simulink model "voltage_isochronous_droop_01"  (R2020b)
settings: Solver=VariableStepAuto  StartTime=0.0  StopTime=5  RelTol=1e-3
undefined symbols (not defined in the file): DiscIntNeverNeededParam, droop1, droop2
libraries: fl_lib x14, nesl_utility x9, simulink x1
settings Model: Creator=gdudgeon  LastModifiedBy=gdudgeon

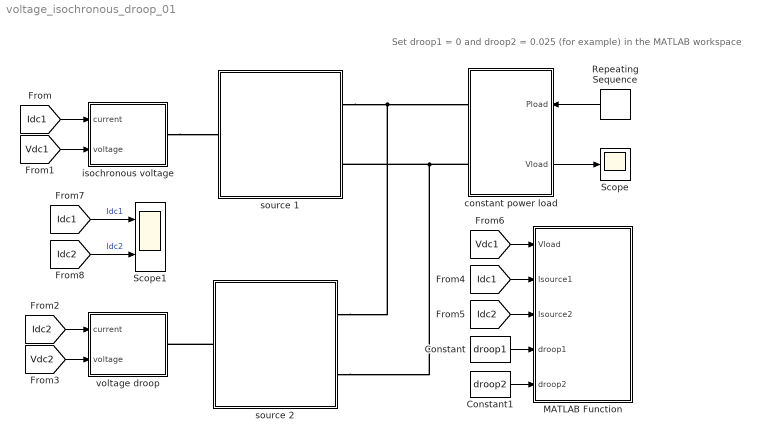
== system voltage_isochronous_droop_01 ==
  note: Set droop1 = 0 and droop2 = 0.025 (for example) in the MATLAB workspace
  Constant : Constant  Value=droop1
  Constant1 : Constant  Value=droop2
  MATLAB Function : MATLAB Function  TreatAsAtomicUnit=on  SystemSampleTime=Tanim  mask(Machine Rotor Animation){Tanim=0.01}
      mask prompts: Tanim "Animation Rate [s]"
      mask help: This block animates permanent magnet inside a stator. The "thetaRotor" input is the angle of the rotor. The "phase" parameter must be defined in the workspace and selects the energized coil in the stator.
  Repeating Sequence : simulink/Sources/Repeating Sequence  rep_seq_t=[0 10 20]  rep_seq_y=[1 1 1]
  Scope : Scope
  Scope1 : Scope  NumInputPorts=2
  constant power load : Subsystem
      settings: PortSchema="{\"entries\":[{\"content\":{\"sides\":[{\"content\":{\"connectorIds\":[\"LConn1\",\"LConn2\"]},\"type\":\"ConnectorPlacement.EquallySpacedRectSide\",\"uuid\":\"ede3b789-4807-48db-8c98-272deebb1f90\"},{\"content\":{\"connectorIds\":[\"In1\",\"Out1\"],\"side\":\"RIGHT\"},\"type\":\"ConnectorPlacement.EquallySpacedRectSide\",\"uuid\":\"cedec5e8-adcb-43e2-ab37-681d5d79ce2a\"},{\"content\":{\"connectorIds\":[],\"side\":\"TOP\"},\"type\":\"ConnectorPlacement.EquallySpacedRectSide\",\"uuid\":\"08b52c53-b13a-4cd2-b8db-308d9ebd4277\"},{\"content\":{\"connectorIds\":[],\"side\":\"HIDDEN\"},\"type\":\"ConnectorPlacement.EquallySpacedRectSide\",\"uuid\":\"3f956204-c540-4879-b053-0f78777aeccb\"}]},\"type\":\"ConnectorPlacement.EquallySpacedConnector\",\"uuid\":\"42303a72-b7ff-4a69-b636-ebca1dcca68c\"}],\"packageUris\":[\"http://schema.mathworks.com/mf0/Connector/R2020b\"],\"version\":\"1.0\"}"
  isochronous voltage : Subsystem  mask{droop=droop1}
  source 1 : Subsystem
  "source 2 " : Subsystem
  voltage droop : Subsystem  mask{droop=droop2}
  wires:
  constant power load/1(Vload) -> Scope/1
  Repeating Sequence/1 -> constant power load/1(Pload)
  Constant/1 -> MATLAB Function/4(droop1)
  Constant1/1 -> MATLAB Function/5(droop2)
  [Idc1] -> isochronous voltage/1(current)
  [Vdc1] -> isochronous voltage/2(voltage)
  [Vdc2] -> voltage droop/2(voltage)
  [Idc2] -> voltage droop/1(current)
  [Idc1] -> MATLAB Function/2(Isource1)
  [Idc2] -> MATLAB Function/3(Isource2)
  [Vdc1] -> MATLAB Function/1(Vload)
  [Idc1] -> Scope1/1  "Idc1"
  [Idc2] -> Scope1/2  "Idc2"
  connections:
  constant power load/LConn2 -- "source 2 "/RConn2 -- source 1/RConn2
  "source 2 "/LConn1 -- voltage droop/RConn1
  source 1/RConn1 -- "source 2 "/RConn1 -- constant power load/LConn1
  isochronous voltage/RConn1 -- source 1/LConn1

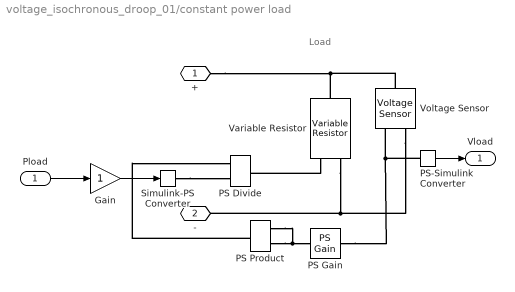
== system voltage_isochronous_droop_01/constant power load ==
  note: Load
  Pload : Inport
  Gain : Gain
  PS Divide : fl_lib/Physical Signals/Functions/PS Divide
      settings: SourceProductBaseCode=SS
  PS Gain : fl_lib/Physical Signals/Functions/PS Gain  gain=-1
  PS Product : fl_lib/Physical Signals/Functions/PS Product
  PS-Simulink Converter : nesl_utility/PS-Simulink Converter  PhysicalDomain=network_engine_domain  SubClassName=ps_output  LeftPortType=input  RightPortType=output  PseudoPeriodic=off  Frequencies=[]  Unit=inherit  AffineConversion=off
  Simulink-PS Converter : nesl_utility/Simulink-PS Converter  PhysicalDomain=network_engine_domain  SubClassName=ps_input  LeftPortType=input  RightPortType=output  PseudoPeriodic=off  Frequencies=[]  NoiseDistribution=none  NoiseParameters=[]  Unit=W  AffineConversion=off  FilteringAndDerivatives=provide  SimscapeFilterOrder=1  InputFilterTimeConstant=0.001  UdotUserProvided=0
  Variable Resistor : fl_lib/Electrical/Electrical Elements/Variable Resistor  Rmin=1 Ohm  i_specify=off  i_priority=None  i=0 A  i_nominal_specify=off  i_nominal_unit=A  i_nominal_value=1  v_specify=off  v_priority=None  v=0 V  v_nominal_specify=off  v_nominal_unit=V  v_nominal_value=1
  Voltage Sensor : fl_lib/Electrical/Electrical Sensors/Voltage Sensor
  + : PMIOPort  Side=Left
  - : PMIOPort  Port=2  Side=Left
  Vload : Outport
  wires:
  PS-Simulink Converter/1 -> Vload/1
  Pload/1 -> Gain/1
  Gain/1 -> Simulink-PS Converter/1
  connections:
  PS-Simulink Converter/LConn1 -- PS Gain/LConn1 -- Voltage Sensor/RConn1
  Variable Resistor/LConn1 -- PS Divide/RConn1
  Voltage Sensor/RConn2 -- -/RConn1 -- Variable Resistor/LConn2
  Voltage Sensor/LConn1 -- +/RConn1 -- Variable Resistor/RConn1
  Simulink-PS Converter/RConn1 -- PS Divide/LConn2
  PS Product/LConn1 -- PS Product/LConn2 -- PS Gain/RConn1
  PS Product/RConn1 -- PS Divide/LConn1

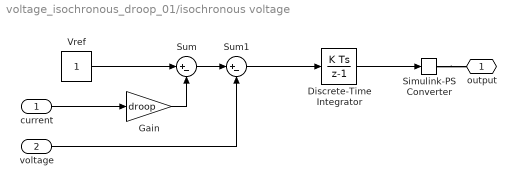
== system voltage_isochronous_droop_01/isochronous voltage ==
  current : Inport
  voltage : Inport  Port=2
  Discrete-Time Integrator : DiscreteIntegrator  gainval=100  InitialCondition=0.5  SampleTime=-1  ICPrevOutput=DiscIntNeverNeededParam  ICPrevScaledInput=DiscIntNeverNeededParam
  Gain : Gain  Gain=droop
  Simulink-PS Converter : nesl_utility/Simulink-PS Converter  PhysicalDomain=network_engine_domain  SubClassName=ps_input  LeftPortType=input  RightPortType=output  PseudoPeriodic=off  Frequencies=[]  NoiseDistribution=none  NoiseParameters=[]  Unit=1  AffineConversion=off  FilteringAndDerivatives=provide  SimscapeFilterOrder=1  InputFilterTimeConstant=0.001  UdotUserProvided=0
  Sum : Sum  Inputs=|+-
  Sum1 : Sum  Inputs=|+-
  Vref : Constant
  output : PMIOPort  Side=Right
  wires:
  voltage/1 -> Sum1/2
  Vref/1 -> Sum/1
  Gain/1 -> Sum/2
  Sum/1 -> Sum1/1
  current/1 -> Gain/1
  Discrete-Time Integrator/1 -> Simulink-PS Converter/1
  Sum1/1 -> Discrete-Time Integrator/1
  connections:
  Simulink-PS Converter/RConn1 -- output/RConn1

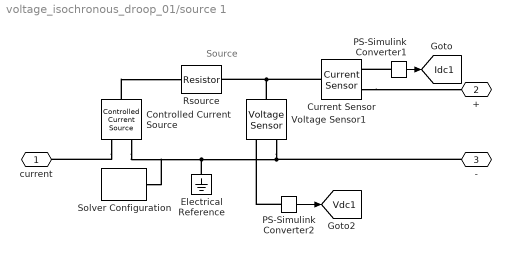
== system voltage_isochronous_droop_01/source 1 ==
  note: Source
  Controlled Current Source : fl_lib/Electrical/Electrical Sources/Controlled Current Source
  Current Sensor : fl_lib/Electrical/Electrical Sensors/Current Sensor
  Electrical Reference : fl_lib/Electrical/Electrical Elements/Electrical Reference
  PS-Simulink Converter1 : nesl_utility/PS-Simulink Converter  PhysicalDomain=network_engine_domain  SubClassName=ps_output  LeftPortType=input  RightPortType=output  PseudoPeriodic=off  Frequencies=[]  Unit=inherit  AffineConversion=off
  PS-Simulink Converter2 : nesl_utility/PS-Simulink Converter  PhysicalDomain=network_engine_domain  SubClassName=ps_output  LeftPortType=input  RightPortType=output  PseudoPeriodic=off  Frequencies=[]  Unit=inherit  AffineConversion=off
  Rsource : fl_lib/Electrical/Electrical Elements/Resistor  R=1e-2 Ohm  i_specify=off  i_priority=None  i=0 A  i_nominal_specify=off  i_nominal_unit=A  i_nominal_value=1  v_specify=off  v_priority=None  v=0 V  v_nominal_specify=off  v_nominal_unit=V  v_nominal_value=1
  Solver Configuration : nesl_utility/Solver Configuration  PhysicalDomain=network_engine_domain  SubClassName=solver  LeftPortType=input  RightPortType=generic  Tones=[]  Harmonics=[]  SimulateNoise=off  Profile=off  UseLocalSampling=off  EnableSwitchedLinearOptims=on  FrequencyDomain=off  UseCCode=off  RelTol=0.001  AbsTol=1e-06  MinStep=1e-09  ToWorkspace=off  RevertToSquareIcSolve=off  NumHomotopyIterations=100  PhasorMode=off  PhasorModeNumHarmonics=1  DoDC=off  ResidualTolerance=1e-09  UseLocalSolver=on  LocalSolverChoice=NE_BACKWARD_EULER_ADVANCER  LocalSolverSampleTime=5e-5  DoFixedCost=on  MaxNonlinIter=3  MaxModeIter=2  ComputeImpulses=off  ImpulseIterations=2  LinearAlgebra=auto  EquationFormulation=NE_TIME_EF  DelaysMemoryBudget=1024  AutomaticFiltering=on  FilteringTimeConstant=0.001  PartitionStorageMethod=AS_NEEDED  PartitionMemoryBudget=1024  PartitionMethod=ROBUST
  Voltage Sensor1 : fl_lib/Electrical/Electrical Sensors/Voltage Sensor
  current : PMIOPort  Side=Left
  "+ " : PMIOPort  Port=2  Side=Right
  "- " : PMIOPort  Port=3  Side=Right
  tag scope: Idc1=global, Vdc1=global
  wires:
  PS-Simulink Converter2/1 -> [Vdc1]
  PS-Simulink Converter1/1 -> [Idc1]
  connections:
  Current Sensor/RConn2 -- "+ "/RConn1
  PS-Simulink Converter1/LConn1 -- Current Sensor/RConn1
  Voltage Sensor1/RConn2 -- Electrical Reference/LConn1 -- Controlled Current Source/RConn2 -- Solver Configuration/RConn1 -- "- "/RConn1
  Controlled Current Source/LConn1 -- Rsource/LConn1
  Current Sensor/LConn1 -- Voltage Sensor1/LConn1 -- Rsource/RConn1
  PS-Simulink Converter2/LConn1 -- Voltage Sensor1/RConn1
  Controlled Current Source/RConn1 -- current/RConn1

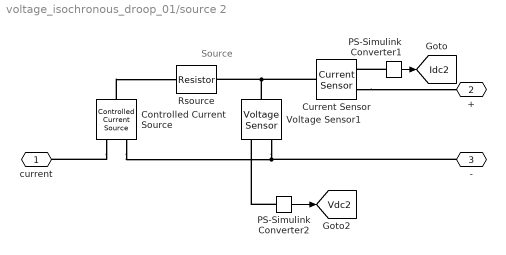
== system voltage_isochronous_droop_01/source 2  ==
  note: Source
  Controlled Current Source : fl_lib/Electrical/Electrical Sources/Controlled Current Source
  Current Sensor : fl_lib/Electrical/Electrical Sensors/Current Sensor
  PS-Simulink Converter1 : nesl_utility/PS-Simulink Converter  PhysicalDomain=network_engine_domain  SubClassName=ps_output  LeftPortType=input  RightPortType=output  PseudoPeriodic=off  Frequencies=[]  Unit=inherit  AffineConversion=off
  PS-Simulink Converter2 : nesl_utility/PS-Simulink Converter  PhysicalDomain=network_engine_domain  SubClassName=ps_output  LeftPortType=input  RightPortType=output  PseudoPeriodic=off  Frequencies=[]  Unit=inherit  AffineConversion=off
  Rsource : fl_lib/Electrical/Electrical Elements/Resistor  R=1e-2 Ohm  i_specify=off  i_priority=None  i=0 A  i_nominal_specify=off  i_nominal_unit=A  i_nominal_value=1  v_specify=off  v_priority=None  v=0 V  v_nominal_specify=off  v_nominal_unit=V  v_nominal_value=1
  Voltage Sensor1 : fl_lib/Electrical/Electrical Sensors/Voltage Sensor
  current : PMIOPort  Side=Left
  "+ " : PMIOPort  Port=2  Side=Right
  "- " : PMIOPort  Port=3  Side=Right
  tag scope: Idc2=global, Vdc2=global
  wires:
  PS-Simulink Converter1/1 -> [Idc2]
  PS-Simulink Converter2/1 -> [Vdc2]
  connections:
  Controlled Current Source/RConn1 -- current/RConn1
  PS-Simulink Converter2/LConn1 -- Voltage Sensor1/RConn1
  Voltage Sensor1/LConn1 -- Rsource/RConn1 -- Current Sensor/LConn1
  Controlled Current Source/LConn1 -- Rsource/LConn1
  "- "/RConn1 -- Controlled Current Source/RConn2 -- Voltage Sensor1/RConn2
  PS-Simulink Converter1/LConn1 -- Current Sensor/RConn1
  Current Sensor/RConn2 -- "+ "/RConn1

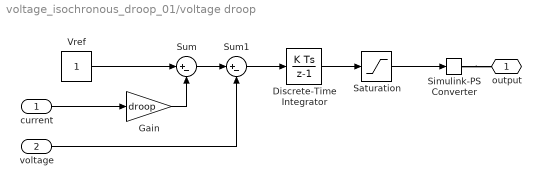
== system voltage_isochronous_droop_01/voltage droop ==
  current : Inport
  voltage : Inport  Port=2
  Discrete-Time Integrator : DiscreteIntegrator  gainval=100  InitialCondition=0.5  SampleTime=-1  ICPrevOutput=DiscIntNeverNeededParam  ICPrevScaledInput=DiscIntNeverNeededParam
  Gain : Gain  Gain=droop
  Saturation : Saturate  UpperLimit=1  LowerLimit=0
  Simulink-PS Converter : nesl_utility/Simulink-PS Converter  PhysicalDomain=network_engine_domain  SubClassName=ps_input  LeftPortType=input  RightPortType=output  PseudoPeriodic=off  Frequencies=[]  NoiseDistribution=none  NoiseParameters=[]  Unit=1  AffineConversion=off  FilteringAndDerivatives=provide  SimscapeFilterOrder=1  InputFilterTimeConstant=0.001  UdotUserProvided=0
  Sum : Sum  Inputs=|+-
  Sum1 : Sum  Inputs=|+-
  Vref : Constant
  output : PMIOPort  Side=Right
  wires:
  Sum/1 -> Sum1/1
  Gain/1 -> Sum/2
  Vref/1 -> Sum/1
  Discrete-Time Integrator/1 -> Saturation/1
  voltage/1 -> Sum1/2
  current/1 -> Gain/1
  Sum1/1 -> Discrete-Time Integrator/1
  Saturation/1 -> Simulink-PS Converter/1
  connections:
  Simulink-PS Converter/RConn1 -- output/RConn1

== matlab function voltage_isochronous_droop_01/MATLAB Function ==
  data: Vload input; Isource1 input; Isource2 input; droop1 input; droop2 input
function plotDroop2(Vload,Isource1,Isource2,droop1,droop2)

persistent hf hp hp2 hp3


if isempty(hf)
    
    figure(1); clf(1); hold on;
    
    [hf,hp,hp2,hp3] = plotBackground(Vload,Isource1,Isource2,droop1,droop2);
  
    drawnow
    
else
    
    updateAnimation(hp,hp2,hp3,Vload,Isource1,Isource2);

    drawnow

end

end


function [hf,hp,hp2,hp3] = plotBackground(Vload,Isource1,Isource2,droop1,droop2)

hf = figure(1);hold on,grid %#ok<*DUALC>

hp = plot([0 1],[1 1]*Vload);xlabel('Power (pu)'),ylabel('Voltage (pu)')
hp2 = plot([1 1]*Isource1*Vload,[0.94 Vload],'k--');

hp3 = plot([1 1]*Isource2*Vload,[0.94 Vload],'k--');

plot([0 1],[1 1-droop1],'r');
plot([0 1],[1 1-droop2],'g');

coder.extrinsic('num2str')

title(['Droop1 = ',num2str(droop1),' : Droop2 = ',num2str(droop2)])


end

function  updateAnimation(hp,hp2,hp3,Vload,Isource1,Isource2)


set(hp,'YData',[1 1]*Vload);

set(hp2,'XData',[1 1]*Isource1*Vload);
set(hp2,'YData',[0.94 Vload]);

set(hp3,'XData',[1 1]*Isource2*Vload);
set(hp3,'YData',[0.94 Vload]);


end
